simulink model "car_model_FIXED"  (R2022b)
settings: Solver=VariableStepAuto  StartTime=0.0  StopTime=60  RelTol=1e-3
values from neighbouring files (symbols this model uses):
  ABS_MAX_TORQUE = [25 25 25 25]    [workspace.mat]
  ABS_MAX_TRQ_CMD = 50    [workspace.mat]
  ABS_MIN_TORQUE = [0.01 0.01 0.01 0.01]    [workspace.mat]
  acc_IC = 0    [workspace.mat]
  ACCELERATION_MAX = 30    [workspace.mat]
  ActSuspDutyCycle = 1    [workspace.mat]
  Aeq_left = [0.305756190204 0.308857786592 0.311945941182 0.315020811431 0.318082554689 0.321131328186 0.324167289011 0.327190594103 0.330201400225 0.333199863958 0.336186141681 0.339160389558 ... (261 elements, 1x261)]    [workspace.mat]
  Aeq_right = [-0.961664782545 -0.959835898365 -0.957982924115 -0.956106413788 -0.954206913862 -0.952284963337 -0.950341093764 -0.948375829284 -0.946389686656 -0.944383175301 -0.942356797333 -0.940311047601 ... (261 elements, 1x261)]    [workspace.mat]
  alpha_error = 0.1    [workspace.mat]
  ang_acc_hystersesis = 0.1    [workspace.mat]
  ang_IC = 0    [workspace.mat]
  ang_vel_IC = 0    [workspace.mat]
  area_air = 0.15    [workspace.mat]
  axb = -5    [workspace.mat]
  battery_current_IC = 0    [workspace.mat]
  BATTERY_CURRENT_MAX = 140    [workspace.mat]
  BATTERY_CURRENT_MIN = 0    [workspace.mat]
  battery_FT_IC = 300    [workspace.mat]
  battery_T_IC = 300    [workspace.mat]
  BATTERY_TEMPERATURE_MAX = 60    [workspace.mat]
  BATTERY_TEMPERATURE_MIN = 0    [workspace.mat]
  battery_voltage_IC = 332    [workspace.mat]
  BATTERY_VOLTAGE_MAX = 340    [workspace.mat]
  BATTERY_VOLTAGE_MIN = 60    [workspace.mat]
  br = 0.01    [workspace.mat]
  brake_bias = [0.35 0.35 0.15 0.15]    [workspace.mat]
  Brake_Pressure_IC = 1    [workspace.mat]
  ccl_IC = 0    [workspace.mat]
  CENTER_STEER_ANGLE_MAX = 130    [workspace.mat]
  covarience_matrix_IC = [0.001 0 0 0 0 0 0 0 0 0 0 0 ... (784 elements, 28x28)]    [workspace.mat]
  CURRENT_BUFFER = 25    [workspace.mat]
  cy_sweep = [13568.4166816 14020.2069783 14456.754831 14879.7402576 15289.7264712 15687.2766846 16072.954111 16447.3219632 16810.9434544 17164.3817975 17508.2002054 17842.9618912 ... (101 elements, 1x101)]    [workspace.mat]
  dB = 0.001    [workspace.mat]
  dcl_IC = 140    [workspace.mat]
  DCL_MAX = 130    [workspace.mat]
  DCL_MIN = 0    [workspace.mat]
  deadband_angle = 12    [workspace.mat]
  dIndex = 50    [workspace.mat]
  driver_t = 0.015    [workspace.mat]
  dt_OFF = 4.5    [workspace.mat]
  dt_ON = 7.5    [workspace.mat]
  dTx = 0.01    [workspace.mat]
  dx = 0.1    [workspace.mat]
  dZ = 0.295    [workspace.mat]
  efficiency_grid = [0.759500051293 0.787587791453 0.809832189108 0.826747821898 0.837164543102 0.842744381136 0.842258400104 0.838611650621 0.82826195101 0.814029316176 0.795690627225 0.7759791486 ... (2782 elements, 26x107)]    [workspace.mat]
  F0z = [0 0]    [workspace.mat]
  forward_look_straight = 5    [workspace.mat]
  forward_look_turn = 15    [workspace.mat]
  Fz_IC = 539.55    [workspace.mat]
  Fz_sweep = [200 210 220 230 240 250 260 270 280 290 300 310 ... (101 elements, 1x101)]    [workspace.mat]
  g = 9.81    [workspace.mat]
  GAIN_ABS = 100    [workspace.mat]
  gearbox_efficiency = [0.8 0.8 0.8 0.8]    [workspace.mat]
  gps_counter_IC = 0    [workspace.mat]
  gps_hz = 0.01    [workspace.mat]
  gr = [8.74786324786 8.74786324786 8.74786324786 8.74786324786]    [workspace.mat]
  I = 0    [workspace.mat]
  I_Driver = 1    [workspace.mat]
  indicies = [3 3.5 4 0.5 1 1.5 2 2.5 3 3.5 4 0.5 ... (27 elements, 1x27)]    [workspace.mat]
  IYY = 0.3    [workspace.mat]
  kx_sweep = [8779.958 9178.302 9576.646 9974.99 10373.334 10771.678 11170.022 11568.366 11966.71 12365.054 12763.398 13161.742 ... (101 elements, 1x101)]    [workspace.mat]
  l = [0.772 0.772]    [workspace.mat]
  lambda_star = 0.15    [workspace.mat]
  low_V_SA = 0.001    [workspace.mat]
  lr = 35    [workspace.mat]
  m_all = 220    [workspace.mat]
  m_body = 180    [workspace.mat]
  m_unsprung = [6 6 14 14]    [workspace.mat]
  MAG_MAX = 200    [workspace.mat]
  Max_Brake_Pressure = 100000000    [workspace.mat]
  Max_Driver_Input = 1    [workspace.mat]
  MAX_DTHETA_DRIVER = 360    [workspace.mat]
  MAX_I_Driver = 1    [workspace.mat]
  MAX_STEERING_ADJUST = 15    [workspace.mat]
  max_yaw = [0.705271610162 0.928228152446 1.12280857731 1.14131008363 1.08727026041 1.01377803859 0.938114723816 0.8718206875 0.815009168116 0.767481919497 0.727119764215 0.694403589394 ... (15 elements, 1x15)]    [workspace.mat]
  Min_Brake_Pressure = 1    [workspace.mat]
  Min_Driver_Input = 0    [workspace.mat]
  min_velocity_regen = 1.4    [workspace.mat]
  motor_current_IC = 0    [workspace.mat]
  MOTOR_CURRENT_MAX = 70    [workspace.mat]
  MOTOR_CURRENT_MIN = 0    [workspace.mat]
  MOTOR_ENABLE = [0 0 1 1]    [workspace.mat]
  motor_FT_IC = 300    [workspace.mat]
  motor_T_IC = 300    [workspace.mat]
  MOTOR_TEMPERATURE_MAX = 100    [workspace.mat]
  MOTOR_TEMPERATURE_MIN = 0    [workspace.mat]
  motor_voltage_IC = 332    [workspace.mat]
  MOTOR_VOLTAGE_MAX = 340    [workspace.mat]
  MOTOR_VOLTAGE_MIN = 90    [workspace.mat]
  motorControllerCurve = [25  260; 50  130; 75  0]    [workspace.mat]
  motorTempCurve = [140 138.6 134.4 127.4 117.6 105 89.6 71.4 50.4 26.6 0]    [workspace.mat]
  motorTempX = [75 77 79 81 83 85 87 89 91 93 95]    [workspace.mat]
  mu_star = 0.5    [workspace.mat]
  mx_sweep = [3.38348 3.3655067 3.3477908 3.3303323 3.3131312 3.2961875 3.2795012 3.2630723 3.2469008 3.2309867 3.21533 3.1999307 ... (101 elements, 1x101)]    [workspace.mat]
  my_sweep = [3.036232 3.015241699 2.994987032 2.975452753 2.956623616 2.938484375 2.921019784 2.904214597 2.888053568 2.872521451 2.857603 2.843282969 ... (101 elements, 1x101)]    [workspace.mat]
  noise_state = [1e-06 1e-06 1e-06 1e-06 0.005 0.005 0.005 1e-06 1e-06 1e-06 1e-06 1e-06 ... (28 elements, 28x1)]    [workspace.mat]
  omega_IC = 0    [workspace.mat]
  OMEGA_MAX = 150    [workspace.mat]
  OMEGA_MIN = 0    [workspace.mat]
  ORIENTATION_MAX = 360    [workspace.mat]
  P = 2    [workspace.mat]
  P_Driver = 0.7    [workspace.mat]
  P_High_Speed = 0.1    [workspace.mat]
  P_Steering_Adjust = 2    [workspace.mat]
  P_Straight_Adjust = 5    [workspace.mat]
  pos_IC = 0    [workspace.mat]
  POS_MAX = 300    [workspace.mat]
  q_thresh = 0.3    [workspace.mat]
  RE = 0.223    [workspace.mat]
  rho = 1.225    [workspace.mat]
  s = [0.649 0.621]    [workspace.mat]
  selected_maxvm = [49.86390724 16.21289794 8.219813569 8.05215527 7.103352929 8.35634983 13.87515039 8.72402841 22.75224945 36.67909339 19.32001297 25.09036962 ... (63 elements, 21x3)]    [workspace.mat]
  selected_sweep = [3 3 3 3 3 3 3 3 3 3 3 3 ... (1288 elements, 644x2)]    [workspace.mat]
  selected_track = [inf inf inf inf inf inf inf inf inf inf inf inf ... (37971 elements, 4219x9)]    [workspace.mat]
  shock_length_IC = 0.1    [workspace.mat]
  SHOCK_LENGTH_MAX = 0.25    [workspace.mat]
  SHOCK_LENGTH_MIN = 0    [workspace.mat]
  state_IC = [1 0 0 0 0 0 0 0 0 0 0 0 ... (28 elements, 28x1)]    [workspace.mat]
  steering_sweep = [0 5 10 15 20 25 30 35 40 45 50 55 ... (27 elements, 1x27)]    [workspace.mat]
  steering_Up_Grid = [0.551231966244 8.36038106007 16.1333806643 23.9559539118 31.8240691982 39.7561724339 47.7157531433 55.7845698794 64.1341708168 73.0798046026 82.7903081349 93.1297322155 ... (615 elements, 41x15)]    [workspace.mat]
  ... (+25 more)
undefined symbols (not defined in the file or in its folder): ax, ay, az, covA, covG, covM, covP, covV, DiscIntNeverNeededParam, fusion_t, fusion_t_sim, gps_ratio, IMU_accel, IMU_gyro, imu_hz, IMU_mag, location_lla_IC, p, phi, psi, q, r, sus, theta, trn, veh, VEH, whl, X, Xdot, Y, Ydot, Z, Zdot
libraries: fl_lib x82, nesl_utility x32, vehdynlibtire x10, vehdynlibsuspension x8, simulink x5, autolibutils x5, sharedtransform x5, sdl_lib x4, EngineCoolingComponents_lib x4, slpidlib x3, SimscapeFluids_lib x3, shared6dof x2
(part 5 of 14)

== system car_model_FIXED/Driver & Environment/Longitudinal Control/ABS ==
  Vx : Inport
  omega : Inport  Port=2
  ABS_ENABLE : Inport  Port=3
  ABS system : Subsystem
  Extremum Seeking Control : slctrlblks/Extremum Seeking Control  timeDomainStatus=Discrete time  SampleTime=driver_t  IntegratorMethods=Backward Euler  paramCount=N  initialVal=IC  omega=omega_force  gain=lr  demodAmp=a  demodPhase=phi_1  modAmp=b  modPhase=phi_2  highPassEnable=on  highPassCutoff=omega_hpf  lowPassEnable=on  lowPassCutoff=omega_lpf  estimatedVarOn=off  HPFFreq=-0.99253  LPFFreq=-0.98511  SampleTimeVar=0.015
  Gain6 : Gain  Gain=GAIN_ABS*brake_bias
  Sum : Sum  Inputs=+
  Unit Delay : UnitDelay  SampleTime=-1  HasFrameUpgradeWarning=on
  Bx : Outport
  OFF_FLAG : Outport  Port=2
  wires:
  ABS system/1(mu) -> Unit Delay/1
  Extremum Seeking Control/1 -> ABS system/1(lambda0)
  Vx/1 -> ABS system/2(Vx)
  omega/1 -> ABS system/3(omega)
  ABS system/3(OFF_FLAG) -> OFF_FLAG/1
  ABS system/2(Bx) -> Sum/1
  ABS_ENABLE/1 -> ABS system/4(ABS_ENABLE)
  Sum/1 -> Gain6/1
  Gain6/1 -> Bx/1
  Unit Delay/1 -> Extremum Seeking Control/1

== system car_model_FIXED/Driver & Environment/Reference Generator/Subsystem ==
  <psi> : Inport
  Constant1 : Constant  Value=2*pi
  Constant2 : Constant  Value=pi
  Constant3 : Constant  Value=-pi
  Constant4 : Constant  Value=2*pi
  Constant5 : Constant  Value=-2*pi
  GreaterThan : RelationalOperator  Operator=>  OutDataTypeStr=boolean  RndMeth=Simplest  InputSameDT=off
  Less Than : RelationalOperator  Operator=<  OutDataTypeStr=boolean  RndMeth=Simplest  InputSameDT=off
  Mod : Math  Operator=mod
  Product : Product
  Product1 : Product
  Sum : Sum  Inputs=+++
  psi_rev : Outport
  wires:
  Product1/1 -> Sum/3
  Less Than/1 -> Product1/2
  GreaterThan/1 -> Product/1
  Mod/1 -> GreaterThan/1, Sum/1, Less Than/1
  Constant1/1 -> Mod/2
  Constant5/1 -> Product/2
  Constant3/1 -> Less Than/2
  Constant4/1 -> Product1/1
  Constant2/1 -> GreaterThan/2
  Product/1 -> Sum/2
  Sum/1 -> psi_rev/1
  <psi>/1 -> Mod/1

== system car_model_FIXED/Vehicle Model/Electronics/360_180 ==
  <psi> : Inport
  Constant1 : Constant  Value=2*pi
  Constant2 : Constant  Value=pi
  Constant3 : Constant  Value=-pi
  Constant4 : Constant  Value=2*pi
  Constant5 : Constant  Value=-2*pi
  GreaterThan : RelationalOperator  Operator=>  OutDataTypeStr=boolean  RndMeth=Simplest  InputSameDT=off
  Less Than : RelationalOperator  Operator=<  OutDataTypeStr=boolean  RndMeth=Simplest  InputSameDT=off
  Mod : Math  Operator=mod
  Product : Product
  Product1 : Product
  Sum : Sum  Inputs=+++
  psi_rev : Outport
  wires:
  Product1/1 -> Sum/3
  Less Than/1 -> Product1/2
  GreaterThan/1 -> Product/1
  Mod/1 -> GreaterThan/1, Sum/1, Less Than/1
  Constant1/1 -> Mod/2
  Constant5/1 -> Product/2
  Constant3/1 -> Less Than/2
  Constant4/1 -> Product1/1
  Constant2/1 -> GreaterThan/2
  Product/1 -> Sum/2
  Sum/1 -> psi_rev/1
  <psi>/1 -> Mod/1

== system car_model_FIXED/Vehicle Model/Electronics/Cooling Sensors ==
  <motor_temperature> : Inport
  <mc_temp> : Inport  Port=2
  <motor_fluid_temperature> : Inport  Port=3
  <battery_temperature> : Inport  Port=4
  <battery_fluid_temperature> : Inport  Port=5
  motor_temperature : Outport
  mc_temp : Outport  Port=2
  motor_fluid_temperature : Outport  Port=3
  battery_temperature : Outport  Port=4
  battery_fluid_temperature : Outport  Port=5
  wires:
  <motor_temperature>/1 -> motor_temperature/1
  <motor_fluid_temperature>/1 -> motor_fluid_temperature/1
  <battery_temperature>/1 -> battery_temperature/1
  <battery_fluid_temperature>/1 -> battery_fluid_temperature/1
  <mc_temp>/1 -> mc_temp/1

== system car_model_FIXED/Vehicle Model/Electronics/Corner Dynamics Sensors ==
  <omega> : Inport
  <steering_angle> : Inport  Port=2
  <shock_length> : Inport  Port=3
  <Fz> : Inport  Port=4
  Transpose : Math  Operator=transpose
  omega : Outport
  steering_angle : Outport  Port=2
  shock_length : Outport  Port=3
  Fz : Outport  Port=4
  wires:
  Transpose/1 -> omega/1  "omega"
  <omega>/1 -> Transpose/1
  <steering_angle>/1 -> steering_angle/1
  <shock_length>/1 -> shock_length/1
  <Fz>/1 -> Fz/1

== system car_model_FIXED/Vehicle Model/Electronics/Navigation Sensors ==
  <chassis_velocity> : Inport  PortDimensions=[1 3]
  <chassis_position> : Inport  Port=2  PortDimensions=[1 3]
  <chassis_acceleration> : Inport  Port=3  PortDimensions=[1 3]
  <chassis_orientation> : Inport  Port=4  PortDimensions=[1 3]
  <chassis_angular_velocity> : Inport  Port=5  PortDimensions=[1 3]
  Bus Creator : BusCreator  Inputs=IMU_accel,IMU_gyro,IMU_mag
  Bus Creator1 : BusCreator  Inputs=2
  GPS : sensorgpslib/GPS  DispRefFrame=NED  PositionInputFormat=Local  ReferenceLocation=location_lla_IC  HorizontalPositionAccuracy=GPS_Z_ACCURACY  VerticalPositionAccuracy=GPS_XY_ACCURACY  VelocityAccuracy=GPS_V_ACCURACY  DecayFactor=GPS_NOISE_FACTOR  SeedDouble=r_GPS  SimulateUsing=Interpreted execution
      settings: LibrarySourceBlock=mspsensorlib/GPS
  IMU : mspsensorlib/IMU  DispRefFrame=NED  Temperature=25  MagneticFieldNED=mag_field_IC  MagneticFieldENU=[ -2.4169, 27.5550, 16.0849 ]  SeedDouble=r_IMU  SimulateUsing=Interpreted execution  AccelParamsMeasurementRange=ACC_MAX  AccelParamsResolution=ACC_RES  AccelParamsConstantBias=ACC_BIAS  AccelParamsAxesMisalignment=ACC_SKEW  AccelParamsNoiseDensity=ACC_VEL_WALK  AccelParamsBiasInstability=ACC_BIAS_INSTABILITY  AccelParamsRandomWalk=ACC_WALK  AccelParamsTemperatureBias=ACC_T_BIAS  AccelParamsTemperatureScaleFactor=ACC_T_SCALE  GyroParamsMeasurementRange=GYR_MAX  GyroParamsResolution=GYR_RES  GyroParamsConstantBias=GYR_BIAS  GyroParamsAxesMisalignment=GYR_SKEW  GyroParamsAccelerationBias=GYR_ACC_BIAS  GyroParamsNoiseDensity=GYR_ANG_WALK  GyroParamsBiasInstability=GYR_BIAS_INSTABILITY  GyroParamsRandomWalk=GYR_WALK  GyroParamsTemperatureBias=GYR_T_BIAS  GyroParamsTemperatureScaleFactor=GYR_T_SCALE  MagParamsMeasurementRange=MAG_MAX  MagParamsResolution=MAG_RES  MagParamsConstantBias=MAG_BIAS  MagParamsAxesMisalignment=MAG_SKEW  MagParamsNoiseDensity=MAG_WHITE  MagParamsBiasInstability=MAG_BIAS_INSTABILITY  MagParamsRandomWalk=MAG_WALK  MagParamsTemperatureBias=MAG_T_BIAS  MagParamsTemperatureScaleFactor=MAG_T_SCALE
  To Workspace1 : ToWorkspace  VariableName=Chassis_Orientation  SaveFormat=Timeseries  SampleTime=-1
  To Workspace2 : ToWorkspace  VariableName=IMU_Measurements  SaveFormat=Timeseries  SampleTime=-1
  Transpose : Math  Operator=transpose
  Transpose1 : Math  Operator=transpose
  Transpose2 : Math  Operator=transpose
  VNED to SNED : MATLAB Function  TreatAsAtomicUnit=on
  integrate angvel : MATLAB Function  TreatAsAtomicUnit=on
  vel : Outport  PortDimensions=3
  pos : Outport  Port=2  PortDimensions=3
  acc : Outport  Port=3  PortDimensions=3
  mag : Outport  Port=4  PortDimensions=3
  gyro : Outport  Port=5  PortDimensions=3
  GS : Outport  Port=6
  Course : Outport  Port=7
  wires:
  <chassis_angular_velocity>/1 -> IMU/2  "ang_vel_VNED"
  <chassis_velocity>/1 -> GPS/2  "vel_NED"
  <chassis_acceleration>/1 -> IMU/1  "accel_VNED"
  <chassis_position>/1 -> GPS/1  "pos_NED"
  integrate angvel/1(Orientation_c) -> Bus Creator1/1, IMU/3  "ang_NED"
  GPS/4 -> Course/1  "ang_NE_mag"
  GPS/3 -> GS/1  "vel_NE_mag"
  GPS/2 -> vel/1  "vel_NED"
  GPS/1 -> pos/1  "pos_LLA"
  VNED to SNED/2(gyro_SNED) -> gyro/1  "gyro_SNED"
  VNED to SNED/1(accel_SNED) -> acc/1  "accel_SNED"
  VNED to SNED/3(mag_SNED) -> mag/1  "mag_SNED"
  <chassis_orientation>/1 -> integrate angvel/1("Orientation_e ")  "ang_NED"
  Transpose2/1 -> Bus Creator/3, VNED to SNED/3(mag_VNED)  "IMU_mag"
  Transpose1/1 -> Bus Creator/2, VNED to SNED/2(gyro_VNED)  "IMU_gyro"
  Transpose/1 -> Bus Creator/1, VNED to SNED/1(accel_VNED)  "IMU_accel"
  IMU/3 -> Transpose2/1
  IMU/1 -> Transpose/1
  IMU/2 -> Transpose1/1
  Bus Creator/1 -> To Workspace2/1
  Bus Creator1/1 -> To Workspace1/1
  integrate angvel/2(Orientation_e) -> Bus Creator1/2  "ang_euler_NED"

== system car_model_FIXED/Vehicle Model/Electronics/Power Sensors ==
  <battery_voltage> : Inport
  <battery_current> : Inport  Port=2
  <motor_voltage> : Inport  Port=3
  <motor_current> : Inport  Port=4
  <power_limits> : Inport  Port=5
  battery_voltage : Outport
  battery_current : Outport  Port=2
  motor_voltage : Outport  Port=3
  motor_current : Outport  Port=4
  power_limits : Outport  Port=5
  wires:
  <battery_voltage>/1 -> battery_voltage/1
  <battery_current>/1 -> battery_current/1
  <motor_voltage>/1 -> motor_voltage/1
  <power_limits>/1 -> power_limits/1
  <motor_current>/1 -> motor_current/1

== system car_model_FIXED/Vehicle Model/Powertrain/Battery Cooling Loop ==
  omega_m : Inport
  Battery_V : Inport  Port=2
  Battery_I : Inport  Port=3
  CL Battery Fans : Inport  Port=4
  CL Battery Pump : Inport  Port=5
  Vg : Inport  Port=6
  Battery Temperature : Outport
  Battery Fluid Temperature : Outport  Port=2

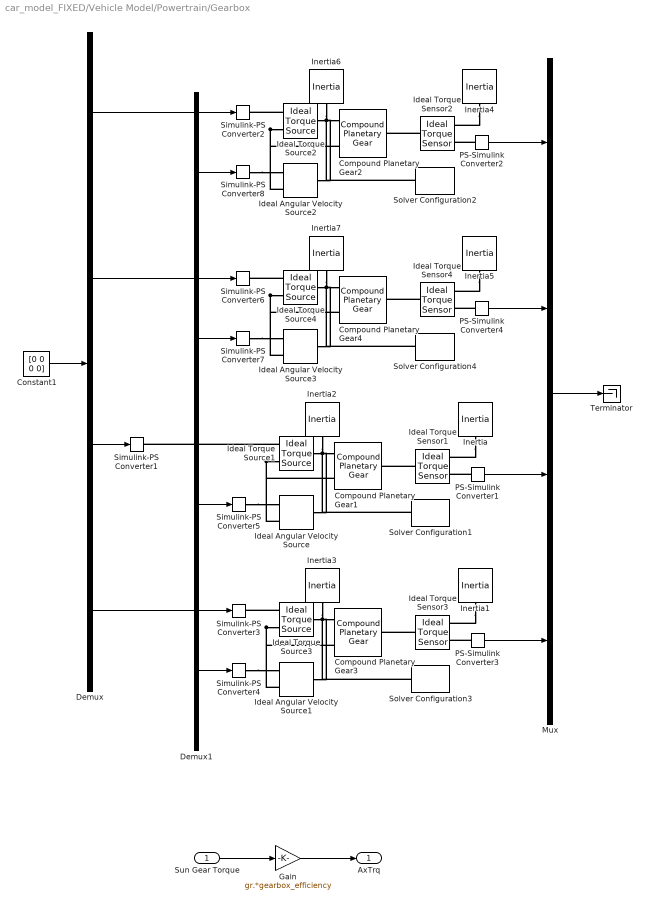
== system car_model_FIXED/Vehicle Model/Powertrain/Gearbox ==
  Sun Gear Torque : Inport
  Compound Planetary Gear{1..4} (4 alike) : sdl_lib/Gears/Compound Planetary Gear  rp_ratio=84/23  ps_ratio=40/21  friction_model=sdl.enum.gear_friction.constant  efficiency=[.97, 1]  temperature_TLU=[280, 300, 320] K  efficiency_sp_TLU=[.95, .9, .85]  efficiency_rp_TLU=[.95, .9, .85]  pwr_thr=[.001, .001] W  mu_visc=[0, 0] N*m/(rad/s)  model_inertia=simscape.enum.onoff.on  planet_inertia=0.001 kg*m^2  thermal_mass=50 J/K  T_init=300 K
      settings: InternalSimscapePortConfiguration="{\"Bottom\":[],\"Left\":[{\"id\":\"C\",\"label\":\"C\",\"type\":\"foundation.mechanical.rotational.rotational\"}],\"Right\":[{\"id\":\"R\",\"label\":\"R\",\"type\":\"foundation.mechanical.rotational.rotational\"},{\"id\":\"S\",\"label\":\"S\",\"type\":\"foundation.mechanical.rotational.rotational\"}],\"Top\":[]}"
  Constant1 : Constant  Value=[0 0 0 0]
  Demux : Demux
  Demux1 : Demux
  Gain : Gain  Gain=gr.*gearbox_efficiency
  Ideal Angular Velocity Source{,1..3} (4 alike) : fl_lib/Mechanical/Mechanical Sources/Ideal Angular Velocity Source
  Ideal Torque Sensor{1..4} (4 alike) : fl_lib/Mechanical/Mechanical Sensors/Ideal Torque Sensor
  Ideal Torque Source{1..4} (4 alike) : fl_lib/Mechanical/Mechanical Sources/Ideal Torque Source
  Inertia{,1,4..5} (4 alike) : fl_lib/Mechanical/Rotational Elements/Inertia  inertia=0.01 kg*m^2  num_ports=foundation.enum.numPorts2.one  w_specify=off  w_priority=High  w=0 rad/s  w_nominal_specify=off  w_nominal_unit=rad/s  w_nominal_value=1  t_specify=off  t_priority=None  t=0 N*m  t_nominal_specify=off  t_nominal_unit=N*m  t_nominal_value=1
  Inertia{2..3,6..7} (4 alike) : fl_lib/Mechanical/Rotational Elements/Inertia  inertia=0.01 kg*m^2  num_ports=foundation.enum.numPorts2.one  w_specify=off  w_priority=High  w=0 rad/s  w_nominal_specify=off  w_nominal_unit=rad/s  w_nominal_value=1  t_specify=on  t_priority=High  t=0 N*m  t_nominal_specify=off  t_nominal_unit=N*m  t_nominal_value=1
  Mux : Mux
  PS-Simulink Converter{1..4} (4 alike) : nesl_utility/PS-Simulink Converter  PhysicalDomain=network_engine_domain  SubClassName=ps_output  LeftPortType=input  RightPortType=output  PseudoPeriodic=off  Frequencies=[]  VectorFormat=1-D array  Unit=inherit  AffineConversion=off
  Simulink-PS Converter{1..3,6} (4 alike) : nesl_utility/Simulink-PS Converter  PhysicalDomain=network_engine_domain  SubClassName=ps_input  LeftPortType=input  RightPortType=output  PseudoPeriodic=off  Frequencies=[]  NoiseDistribution=none  NoiseParameters=[]  Unit=N*m  AffineConversion=off  FilteringAndDerivatives=zero  SimscapeFilterOrder=1  InputFilterTimeConstant=0.001  UdotUserProvided=0
  Simulink-PS Converter{4..5,7..8} (4 alike) : nesl_utility/Simulink-PS Converter  PhysicalDomain=network_engine_domain  SubClassName=ps_input  LeftPortType=input  RightPortType=output  PseudoPeriodic=off  Frequencies=[]  NoiseDistribution=none  NoiseParameters=[]  Unit=rad/s  AffineConversion=off  FilteringAndDerivatives=zero  SimscapeFilterOrder=1  InputFilterTimeConstant=0.001  UdotUserProvided=0
  Solver Configuration{1..4} (4 alike) : nesl_utility/Solver Configuration  PhysicalDomain=network_engine_domain  SubClassName=solver  LeftPortType=input  RightPortType=generic  Tones=[]  Harmonics=[]  SimulateNoise=off  Profile=off  UseLocalSampling=off  EnableSwitchedLinearOptims=on  FrequencyDomain=off  UseCCode=off  RelTol=0.001  AbsTol=1e-06  MinStep=1e-09  ToWorkspace=off  RevertToSquareIcSolve=off  NumHomotopyIterations=100  PhasorMode=off  PhasorModeNumHarmonics=1  ConsistencySolver=NEWTON_FTOL  IndexReductionMethod=DerivativeReplacement  DoDC=off  ResidualTolerance=1e-09  ConsistencyTolSource=GLOBAL  ConsistencyAbsTol=0.001  ConsistencyRelTol=0.001  ConsistencyTolFactor=0.001  UseLocalSolver=off  LocalSolverChoice=NE_BACKWARD_EULER_ADVANCER  ResolveIndetEquations=on  FunctionEvalNumThread=1  LocalSolverSampleTime=0.000001  DoFixedCost=off  MaxNonlinIter=300  MaxModeIter=2  ComputeImpulses=off  ImpulseIterations=2  LinearAlgebra=auto  LinearAlgebraNumThread=0  EquationFormulation=NE_TIME_EF  DelaysMemoryBudget=1024  AutomaticFiltering=off  FilteringTimeConstant=0.001  PartitionStorageMethod=AS_NEEDED  PartitionMemoryBudget=1024  PartitionMethod=ROBUST
  Terminator : Terminator
  AxTrq : Outport  PortDimensions=[1 4]
  wires:
  Demux/2 -> Simulink-PS Converter6/1
  Demux/3 -> Simulink-PS Converter1/1
  Demux/1 -> Simulink-PS Converter2/1
  Constant1/1 -> Demux/1
  Mux/1 -> Terminator/1
  PS-Simulink Converter1/1 -> Mux/3
  Demux1/3 -> Simulink-PS Converter5/1
  PS-Simulink Converter3/1 -> Mux/4
  Demux/4 -> Simulink-PS Converter3/1
  Demux1/4 -> Simulink-PS Converter4/1
  PS-Simulink Converter2/1 -> Mux/1
  Demux1/1 -> Simulink-PS Converter8/1
  Demux1/2 -> Simulink-PS Converter7/1
  PS-Simulink Converter4/1 -> Mux/2
  ? -> Demux1/1
  Sun Gear Torque/1 -> Gain/1
  Gain/1 -> AxTrq/1
  connections:
  Compound Planetary Gear1/RConn2 -- Ideal Angular Velocity Source/LConn1 -- Solver Configuration1/RConn1 -- Ideal Torque Source1/LConn1 -- Inertia2/LConn1
  Ideal Torque Source1/RConn2 -- Ideal Angular Velocity Source/RConn2 -- Compound Planetary Gear1/RConn1
  Inertia/LConn1 -- Ideal Torque Sensor1/RConn1
  Ideal Torque Sensor1/LConn1 -- Compound Planetary Gear1/LConn1
  PS-Simulink Converter1/LConn1 -- Ideal Torque Sensor1/RConn2
  Simulink-PS Converter5/RConn1 -- Ideal Angular Velocity Source/RConn1
  Ideal Torque Source1/RConn1 -- Simulink-PS Converter1/RConn1
  Compound Planetary Gear3/RConn2 -- Ideal Angular Velocity Source1/LConn1 -- Solver Configuration3/RConn1 -- Ideal Torque Source3/LConn1 -- Inertia3/LConn1
  Ideal Torque Source3/RConn2 -- Ideal Angular Velocity Source1/RConn2 -- Compound Planetary Gear3/RConn1
  Inertia1/LConn1 -- Ideal Torque Sensor3/RConn1
  Ideal Torque Sensor3/LConn1 -- Compound Planetary Gear3/LConn1
  PS-Simulink Converter3/LConn1 -- Ideal Torque Sensor3/RConn2
  Simulink-PS Converter4/RConn1 -- Ideal Angular Velocity Source1/RConn1
  Ideal Torque Source3/RConn1 -- Simulink-PS Converter3/RConn1
  Ideal Torque Source4/RConn2 -- Ideal Angular Velocity Source3/RConn2 -- Compound Planetary Gear4/RConn1
  Ideal Torque Source2/RConn2 -- Ideal Angular Velocity Source2/RConn2 -- Compound Planetary Gear2/RConn1
  Compound Planetary Gear4/RConn2 -- Ideal Angular Velocity Source3/LConn1 -- Solver Configuration4/RConn1 -- Ideal Torque Source4/LConn1 -- Inertia7/LConn1
  Compound Planetary Gear2/RConn2 -- Ideal Angular Velocity Source2/LConn1 -- Solver Configuration2/RConn1 -- Ideal Torque Source2/LConn1 -- Inertia6/LConn1
  Simulink-PS Converter7/RConn1 -- Ideal Angular Velocity Source3/RConn1
  Ideal Torque Source2/RConn1 -- Simulink-PS Converter2/RConn1
  PS-Simulink Converter2/LConn1 -- Ideal Torque Sensor2/RConn2
  Inertia4/LConn1 -- Ideal Torque Sensor2/RConn1
  PS-Simulink Converter4/LConn1 -- Ideal Torque Sensor4/RConn2
  Ideal Torque Source4/RConn1 -- Simulink-PS Converter6/RConn1
  Inertia5/LConn1 -- Ideal Torque Sensor4/RConn1
  Ideal Torque Sensor4/LConn1 -- Compound Planetary Gear4/LConn1
  Simulink-PS Converter8/RConn1 -- Ideal Angular Velocity Source2/RConn1
  Ideal Torque Sensor2/LConn1 -- Compound Planetary Gear2/LConn1
